simulink model "KalmanFilterSim"  (R2017a)
settings: Solver=FixedStepDiscrete  StartTime=0.0  StopTime=3  FixedStep=0.001  RelTol=1e-3
undefined symbols (not defined in the file or in its folder): Discrete, Time
libraries: ctrlSharedLib x4, dspsrcs4 x3, powerlib_meascontrol x2
settings Model: Creator=Danie  LastModifiedBy=Danie

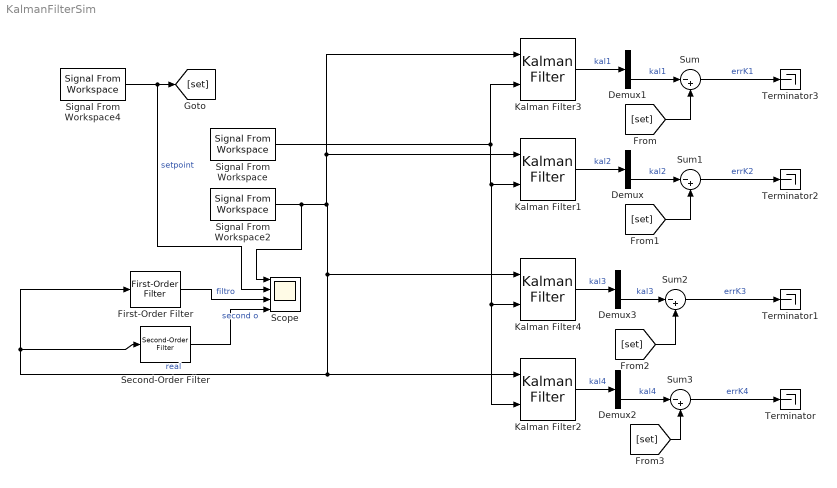
== system KalmanFilterSim ==
  Demux{,1..3} (4 alike) : Demux  Outputs=2
  First-Order Filter : powerlib_meascontrol/Filters/First-Order Filter  FilterType=Lowpass  Tc=10e-3  Ts=0.001  Initialize=on  Vac_Init=[0, 0, 60]  Vdc_Init=0  PlotResponse=off  FreqRange="[0,  200,  1]"
      settings: SourceProductName=Simscape Power Systems
  Kalman Filter1 : ctrlSharedLib/Kalman Filter  TimeDomain=Discrete-Time  UseCurrentEstimator=on  ModelSource=Individual A, B, C, D matrices  ModelSourceVariable=ss(0.95,1,1,0,1)  A=[1 0.001; 0 1]  B=[0 ;0.001]  C=[1 0 ]  D=0  NumberOfStates=1  NumberOfInputs=1  NumberOfOutputs=1  InitialEstimateSource=Dialog  X0=0  P0=10  UseK=off  UseGH=off  NumberOfProcessNoiseInputs=1  G=1  TimeInvariantG=on  H=0  TimeInvariantH=on  Q=[1e-5 0;0 1e-1]  TimeInvariantQ=on  R=1e-3  TimeInvariantR=on  N=0  TimeInvariantN=on  AddInputPort=on  AddEnablePort=off  OutputEstimatedY=off  OutputP=off  Ts=0.001
  Kalman Filter2 : ctrlSharedLib/Kalman Filter  TimeDomain=Discrete-Time  UseCurrentEstimator=on  ModelSource=Individual A, B, C, D matrices  ModelSourceVariable=ss(0.95,1,1,0,1)  A=[1 0.001; 0 1]  B=[0 ;0.001]  C=[1 0 ]  D=0  NumberOfStates=1  NumberOfInputs=1  NumberOfOutputs=1  InitialEstimateSource=Dialog  X0=0  P0=10  UseK=off  UseGH=off  NumberOfProcessNoiseInputs=1  G=1  TimeInvariantG=on  H=0  TimeInvariantH=on  Q=[1e-5 0;0 1e-1]  TimeInvariantQ=on  R=1e-2  TimeInvariantR=on  N=0  TimeInvariantN=on  AddInputPort=on  AddEnablePort=off  OutputEstimatedY=off  OutputP=off  Ts=0.001
  Kalman Filter3 : ctrlSharedLib/Kalman Filter  TimeDomain=Discrete-Time  UseCurrentEstimator=on  ModelSource=Individual A, B, C, D matrices  ModelSourceVariable=ss(0.95,1,1,0,1)  A=[1 0.001; 0 1]  B=[0 ;0.001]  C=[1 0 ]  D=0  NumberOfStates=1  NumberOfInputs=1  NumberOfOutputs=1  InitialEstimateSource=Dialog  X0=0  P0=10  UseK=off  UseGH=off  NumberOfProcessNoiseInputs=1  G=1  TimeInvariantG=on  H=0  TimeInvariantH=on  Q=[0.1 0;0 1000]  TimeInvariantQ=on  R=1e-15  TimeInvariantR=on  N=0  TimeInvariantN=on  AddInputPort=on  AddEnablePort=off  OutputEstimatedY=off  OutputP=off  Ts=0.001
  Kalman Filter4 : ctrlSharedLib/Kalman Filter  TimeDomain=Discrete-Time  UseCurrentEstimator=on  ModelSource=Individual A, B, C, D matrices  ModelSourceVariable=ss(0.95,1,1,0,1)  A=[1 0.001; 0 1]  B=[0 ;0.001]  C=[1 0 ]  D=0  NumberOfStates=1  NumberOfInputs=1  NumberOfOutputs=1  InitialEstimateSource=Dialog  X0=0  P0=10  UseK=off  UseGH=off  NumberOfProcessNoiseInputs=1  G=1  TimeInvariantG=on  H=0  TimeInvariantH=on  Q=[1e-5 0;0 1e-1]  TimeInvariantQ=on  R=1e-7  TimeInvariantR=on  N=0  TimeInvariantN=on  AddInputPort=on  AddEnablePort=off  OutputEstimatedY=off  OutputP=off  Ts=0.001
  Scope : Scope  NumInputPorts=4
  Second-Order Filter : powerlib_meascontrol/Filters/Second-Order Filter  FilterType=Lowpass  Fo=10  Zeta=0.707  Ts=0.001  Initialize=on  Vac_Init="[0,  0,  60]"  Vdc_Init=0  PlotResponse=off  FreqRange=[0, 500, 1]
      settings: SourceProductName=Simscape Power Systems  SourceProductBaseCode=PS
  Signal From Workspace : dspsrcs4/Signal From Workspace  X=theta1R  Ts=0.001  nsamps=1  OutputAfterFinalValue=Setting to zero  ignoreOrWarnInputAndFrameLengths=off  OutputFrames=off
  Signal From Workspace2 : dspsrcs4/Signal From Workspace  X=theta1pR  Ts=0.001  nsamps=1  OutputAfterFinalValue=Setting to zero  ignoreOrWarnInputAndFrameLengths=off  OutputFrames=off
  Signal From Workspace4 : dspsrcs4/Signal From Workspace  X=theta1pS  Ts=0.001  nsamps=1  OutputAfterFinalValue=Setting to zero  ignoreOrWarnInputAndFrameLengths=off  OutputFrames=off
  Sum{,1..3} (4 alike) : Sum  Inputs=|-+
  Terminator{,1..3} (4 alike) : Terminator
  wires:
  Kalman Filter2/1 -> Demux2/1  "kal4"
  Kalman Filter3/1 -> Demux1/1  "kal1"
  Kalman Filter4/1 -> Demux3/1  "kal3"
  Kalman Filter1/1 -> Demux/1  "kal2"
  Signal From Workspace2/1 -> Scope/1, Second-Order Filter/1, First-Order Filter/1, Kalman Filter2/1, Kalman Filter4/1, Kalman Filter1/1, Kalman Filter3/1  "real"
  Signal From Workspace/1 -> Kalman Filter3/2, Kalman Filter2/2, Kalman Filter4/2, Kalman Filter1/2
  Demux1/2 -> Sum/1  "kal1"
  Signal From Workspace4/1 -> Scope/2, [set]  "setpoint"
  [set] -> Sum/2
  [set] -> Sum1/2
  Demux/2 -> Sum1/1  "kal2"
  [set] -> Sum2/2
  Demux3/2 -> Sum2/1  "kal3"
  [set] -> Sum3/2
  Demux2/2 -> Sum3/1  "kal4"
  Sum3/1 -> Terminator/1  "errK4"
  Sum2/1 -> Terminator1/1  "errK3"
  Sum1/1 -> Terminator2/1  "errK2"
  Sum/1 -> Terminator3/1  "errK1"
  Second-Order Filter/1 -> Scope/4  "second o"
  First-Order Filter/1 -> Scope/3  "filtro"
